simulink model "DC_Motor_Single_PI"  (R2021a)
settings: Solver=FixedStepAuto  StartTime=0.0  StopTime=3  FixedStep=1e-4  RelTol=1e-3
values from neighbouring files (symbols this model uses):
  B = 0.002    [motor_params.m]
  J = 0.05    [motor_params.m]
  Ke = 1.5    [motor_params.m]
  Kt = 1.5    [motor_params.m]
  L = 0.02    [motor_params.m]
  R = 2.5    [motor_params.m]
  V_nom = 240    [motor_params.m]
libraries: simulink x1, pid_lib x1
settings Model: Creator=DELL  LastModifiedBy=DELL

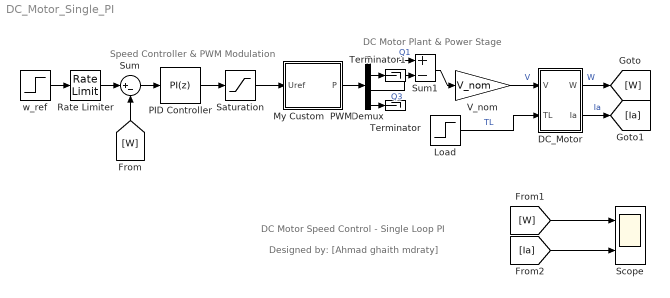
== system DC_Motor_Single_PI ==
  note: Designed by: [Ahmad ghaith mdraty]
  note: DC Motor Speed Control - Single Loop PI
  note: DC Motor Plant & Power Stage
  note: Speed Controller & PWM Modulation
  DC_Motor : Subsystem
  Demux : Demux
  Load : Step  Time=2  Before=1  After=10  SampleTime=0
  My Custom  PWM : Subsystem  mask{PWM_Mode=Unipolar}
      mask prompts: PWM_Mode "Select PWM Modulation:"
      mask TypeOptions PWM_Mode: Bipolar | Unipolar
  PID Controller : pid_lib/PID Controller  Controller=PI  Form=Parallel  TimeDomain=Discrete-time  UseExternalTs=off  SampleTime=-1  IntegratorMethod=Forward Euler  FilterMethod=Forward Euler  ControllerParametersSource=internal  P=0.05  I=2  D=0  UseFilter=on  N=100  TunerSelectOption=Transfer Function Based (PID Tuner App)  InitialConditionSource=internal  InitialConditionForIntegrator=0  InitialConditionForFilter=0  DifferentiatorICPrevScaledInput=0  ExternalReset=none  TrackingMode=off  Kt=1  LimitOutput=off  SatLimitsSource=internal  UpperSaturationLimit=inf  LowerSaturationLimit=-inf  LinearizeAsGain=on  AntiWindupMode=none  Kb=1  POutMin=[]  POutMax=[]  IOutMin=[]  IOutMax=[]  DOutMin=[]  DOutMax=[]  NOutMin=[]  NOutMax=[]  SumOutMin=[]  SumOutMax=[]  SaturationOutMin=[]  SaturationOutMax=[]  PParamMin=[]  PParamMax=[]  IParamMin=[]  IParamMax=[]  DParamMin=[]  DParamMax=[]  NParamMin=[]  NParamMax=[]  KbParamMin=[]  KbParamMax=[]  KtParamMin=[]  KtParamMax=[]  KbOutMin=[]  KbOutMax=[]  KtOutMin=[]  KtOutMax=[]  IntegratorOutMin=[]  IntegratorOutMax=[]  FilterOutMin=[]  FilterOutMax=[]  SumI1OutMin=[]  SumI1OutMax=[]  SumI2OutMin=[]  SumI2OutMax=[]  SumI3OutMin=[]  SumI3OutMax=[]  SumI4OutMin=[]  SumI4OutMax=[]  SumDOutMin=[]  SumDOutMax=[]  DifferentiatorOutMin=[]  DifferentiatorOutMax=[]  FilterDiffOutCoefMin=[]  FilterDiffOutCoefMax=[]  ReciprocalOutMin=[]  ReciprocalOutMax=[]  SumDenOutMin=[]  SumDenOutMax=[]  SumNumOutMin=[]  SumNumOutMax=[]  DivideOutMin=[]  DivideOutMax=[]  UdiffTsProdOutMin=[]  UdiffTsProdOutMax=[]  NTsProdOutMin=[]  NTsProdOutMax=[]  UintegralTsProdOutMin=[]  UintegralTsProdOutMax=[]  UngainTsProdOutMin=[]  UngainTsProdOutMax=[]  IntegratorContinuousStateAttributes=''  IntegratorStateMustResolveToSignalObject=off  IntegratorRTWStateStorageClass=Auto  FilterContinuousStateAttributes=''  FilterStateMustResolveToSignalObject=off  FilterRTWStateStorageClass=Auto  ParallelPVariant=InternalParameters  IdealPVariant=Disabled  IVariant=InternalParameters  DVariant=Disabled  IntegratorVariant=Discrete  SatVariant=Disabled  AWVariant=Passthrough  PCopyVariant=Disabled  TRVariant=Disabled  FdbkBlocksVariant=Forward  IdealPFdbkVariant=Disabled  SatFdbkVariant=Disabled  DerivativeFilterVariant=Disabled  NVariant=Disabled  NCopyVariant=Disabled_SignalSpec  FilterICVariant=Disabled  IntegratorICVariant=InternalICs  ExternalResetVariant=Disabled  TRSumVariant=Passthrough  SumFdbkVariant=Disabled  SumVariant=Sum_PI  TsampFilterVariant=InternalTs  TsampNgainVariant=Passthrough  TsampIntegralVariant=Passthrough  ExternalSaturationOutDataTypeStr=Inherit: Same as second input
  Rate Limiter : RateLimiter  RisingSlewLimit=50  FallingSlewLimit=-50  SampleTimeMode=inherited
  Saturation : Saturate  UpperLimit=1  LowerLimit=-1
  Scope : Scope  NumInputPorts=2
  Sum : Sum  Inputs=|+-
  Sum1 : Sum  Inputs=+-  OutDataTypeStr=double
  Terminator : Terminator
  Terminator1 : Terminator
  V_nom : Gain  Gain=V_nom
  w_ref : Step  Time=0.5  After=50  SampleTime=0
  wires:
  Saturation/1 -> My Custom  PWM/1(Uref)
  PID Controller/1 -> Saturation/1
  Rate Limiter/1 -> Sum/1
  w_ref/1 -> Rate Limiter/1
  Sum/1 -> PID Controller/1
  V_nom/1 -> DC_Motor/1(V)  "V"
  Load/1 -> DC_Motor/2(TL)  "TL"
  My Custom  PWM/1(P) -> Demux/1
  Demux/4 -> Terminator/1
  Demux/1 -> Sum1/1  "Q1"
  Sum1/1 -> V_nom/1
  Demux/2 -> Terminator1/1
  Demux/3 -> Sum1/2  "Q3"
  DC_Motor/1(W) -> [W]  "W"
  [W] -> Sum/2
  DC_Motor/2(Ia) -> [Ia]  "Ia"
  [W] -> Scope/1
  [Ia] -> Scope/2

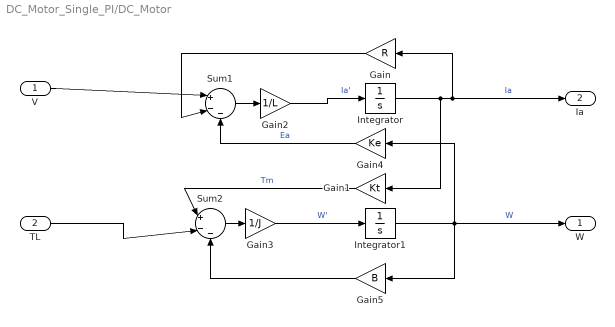
== system DC_Motor_Single_PI/DC_Motor ==
  V : Inport
  TL : Inport  Port=2
  Gain : Gain  Gain=R
  Gain1 : Gain  Gain=Kt
  Gain2 : Gain  Gain=1/L
  Gain3 : Gain  Gain=1/J
  Gain4 : Gain  Gain=Ke
  Gain5 : Gain  Gain=B
  Integrator : Integrator
  Integrator1 : Integrator
  Sum1 : Sum  Inputs=|+--
  Sum2 : Sum  Inputs=|+--
  W : Outport
  Ia : Outport  Port=2
  wires:
  TL/1 -> Sum2/2
  Integrator1/1 -> W/1, Gain5/1, Gain4/1  "W"
  Sum1/1 -> Gain2/1
  Gain/1 -> Sum1/2
  V/1 -> Sum1/1
  Gain5/1 -> Sum2/3
  Gain1/1 -> Sum2/1  "Tm"
  Gain4/1 -> Sum1/3  "Ea"
  Sum2/1 -> Gain3/1
  Integrator/1 -> Gain1/1, Ia/1, Gain/1  "Ia"
  Gain3/1 -> Integrator1/1  "W'"
  Gain2/1 -> Integrator/1  "Ia'"

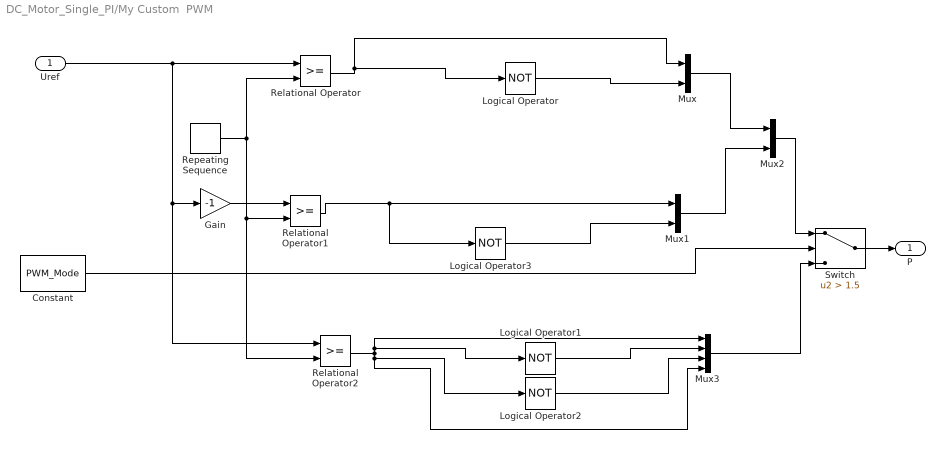
== system DC_Motor_Single_PI/My Custom  PWM ==
  Uref : Inport
  Constant : Constant  Value=PWM_Mode
  Gain : Gain  Gain=-1
  Logical Operator{,1..3} (4 alike) : Logic  Operator=NOT  Inputs=1  AllPortsSameDT=off  OutDataTypeStr=boolean
  Mux : Mux  Inputs=2
  Mux1 : Mux  Inputs=2
  Mux2 : Mux  Inputs=2
  Mux3 : Mux
  Relational Operator : RelationalOperator  OutDataTypeStr=boolean  RndMeth=Simplest
  Relational Operator1 : RelationalOperator  OutDataTypeStr=boolean  RndMeth=Simplest
  Relational Operator2 : RelationalOperator  OutDataTypeStr=boolean  RndMeth=Simplest
  Repeating Sequence : simulink/Sources/Repeating Sequence  rep_seq_t="[0  1/(2*5000)  1/5000]"  rep_seq_y="[-1  1  -1]"
  Switch : Switch  Criteria=u2 > Threshold  Threshold=1.5
  P : Outport
  wires:
  Logical Operator/1 -> Mux/2
  Relational Operator/1 -> Logical Operator/1, Mux/1
  Gain/1 -> Relational Operator1/1
  Uref/1 -> Relational Operator/1, Relational Operator2/1, Gain/1
  Relational Operator1/1 -> Logical Operator3/1, Mux1/1
  Logical Operator3/1 -> Mux1/2
  Mux/1 -> Mux2/1
  Mux1/1 -> Mux2/2
  Logical Operator2/1 -> Mux3/3
  Logical Operator1/1 -> Mux3/2
  Repeating Sequence/1 -> Relational Operator1/2, Relational Operator2/2, Relational Operator/2
  Relational Operator2/1 -> Logical Operator1/1, Mux3/1, Logical Operator2/1, Mux3/4
  Mux3/1 -> Switch/3
  Switch/1 -> P/1
  Mux2/1 -> Switch/1
  Constant/1 -> Switch/2
